simulink model "udpdata"  (R2022a)
settings: Solver=FixedStepAuto  StartTime=0.0  StopTime=10  FixedStep=1  RelTol=1e-3
libraries: etargetslib x1, slrealtimeiplib x1
settings Model: Creator=Pc  LastModifiedBy=Pc

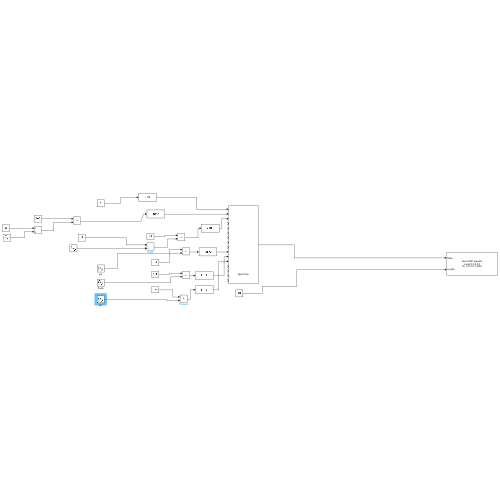
[thumbnail: Simulink's stored preview of the top-level diagram]
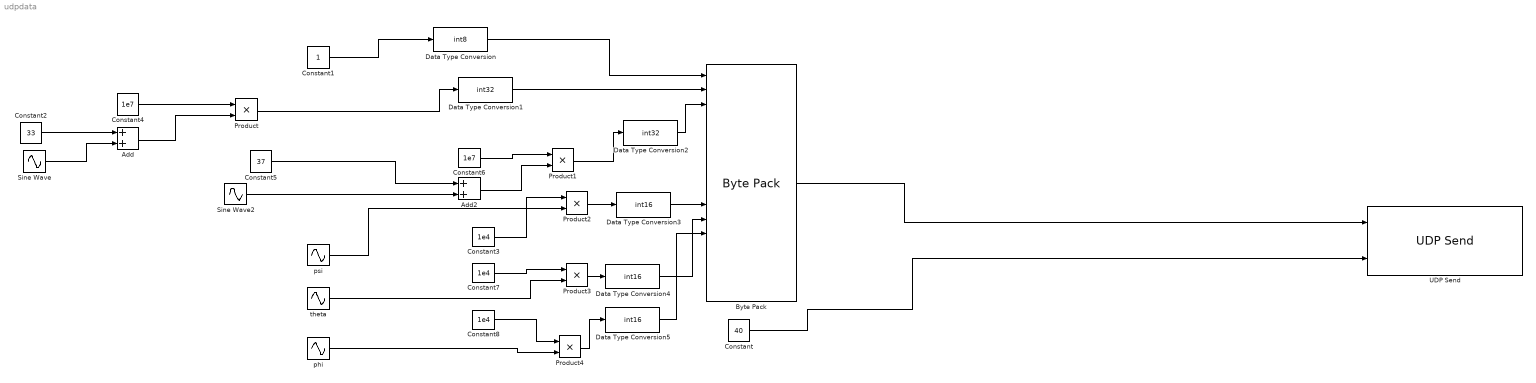
== system udpdata ==
  Add : Sum
  Add2 : Sum
  Byte Pack : etargetslib/Byte Pack  datatypes={'int8','int32','int32','int16','int16','int16','int32','int32','int32','int16','int16','int16','int16','int16','int16','int8'}  byteAlign=1
  Constant : Constant  Value=40
  Constant1 : Constant  OutDataTypeStr=int32
  Constant2 : Constant  Value=33  OutDataTypeStr=int32
  Constant3 : Constant  Value=1e4  OutDataTypeStr=int32
  Constant4 : Constant  Value=1e7  OutDataTypeStr=int32
  Constant5 : Constant  Value=37  OutDataTypeStr=int32
  Constant6 : Constant  Value=1e7  OutDataTypeStr=int32
  Constant7 : Constant  Value=1e4  OutDataTypeStr=int32
  Constant8 : Constant  Value=1e4  OutDataTypeStr=int32
  Data Type Conversion : DataTypeConversion  OutDataTypeStr=int8  SaturateOnIntegerOverflow=off  RndMeth=Floor
  Data Type Conversion1 : DataTypeConversion  OutDataTypeStr=int32  SaturateOnIntegerOverflow=off  RndMeth=Floor
  Data Type Conversion2 : DataTypeConversion  OutDataTypeStr=int32  SaturateOnIntegerOverflow=off  RndMeth=Floor
  Data Type Conversion3 : DataTypeConversion  OutDataTypeStr=int16  SaturateOnIntegerOverflow=off  RndMeth=Floor
  Data Type Conversion4 : DataTypeConversion  OutDataTypeStr=int16  SaturateOnIntegerOverflow=off  RndMeth=Floor
  Data Type Conversion5 : DataTypeConversion  OutDataTypeStr=int16  SaturateOnIntegerOverflow=off  RndMeth=Floor
  Product{,1..4} (5 alike) : Product
  Sine Wave : Sin  Amplitude=10/111e3  SampleTime=0
  Sine Wave2 : Sin  Amplitude=10/111e3  SampleTime=0
  UDP Send : slrealtimeiplib/UDP Send  useHostTargetConn=off  toAddress='127.0.0.1'  toPort=4455  sampleTime=-1  enableMessage=off
      settings: SourceProductBaseCode=XP
  phi : Sin  Amplitude=10/57  SampleTime=0
  psi : Sin  Amplitude=10/57  SampleTime=0
  theta : Sin  Amplitude=10/57  SampleTime=0
  wires:
  Byte Pack/1 -> UDP Send/1
  Constant/1 -> UDP Send/2
  Constant2/1 -> Add/1
  Sine Wave/1 -> Add/2
  Constant1/1 -> Data Type Conversion/1
  Data Type Conversion/1 -> Byte Pack/1
  Add/1 -> Product/2
  Constant4/1 -> Product/1
  Product/1 -> Data Type Conversion1/1
  Sine Wave2/1 -> Add2/2
  Constant6/1 -> Product1/1
  Constant5/1 -> Add2/1
  Add2/1 -> Product1/2
  Product1/1 -> Data Type Conversion2/1
  Constant3/1 -> Product2/1
  psi/1 -> Product2/2
  Product2/1 -> Data Type Conversion3/1
  theta/1 -> Product3/2
  Constant7/1 -> Product3/1
  Product3/1 -> Data Type Conversion4/1
  Constant8/1 -> Product4/1
  Product4/1 -> Data Type Conversion5/1
  phi/1 -> Product4/2
  Data Type Conversion1/1 -> Byte Pack/2
  Data Type Conversion2/1 -> Byte Pack/3
  Data Type Conversion3/1 -> Byte Pack/10
  Data Type Conversion4/1 -> Byte Pack/11
  Data Type Conversion5/1 -> Byte Pack/12
